simulink model "Model_RB_APF_WF_VO_withFairRules"  (R2024b)
settings: Solver=FixedStepAuto  StartTime=0.0  StopTime=150  FixedStep=UAVSampleTime  RelTol=1e-3
undefined symbols (not defined in the file): DroneMass, Gravity, Horizontal_Limits, Horizontal_Res, kD_pos, kD_vel, kI_pos, kI_vel, kP_pos, kP_vel, Lidar, MaxRange, N_filter, TopSpeed, UAV, Vertical_Limits, Vertical_Res, Waypoints
libraries: slpidlib x6, uavsimlib x4, robotcorelib x1, uavalgslib x1
(part 2 of 2)

== matlab function Model_RB_APF_WF_VO_withFairRules/LML Indicators/LML_indicators ==
  settings: updateMethod=DISCRETE
  data: APF_pos input; APF_mag output; position input; target input; disp_1s output; t input; disp_3s output; dist2goal output
function [APF_mag, disp_1s, disp_3s, dist2goal] = LML_indicators(APF_pos, position, target, t)

Tmax = 180;

persistent pos_hist
persistent lastSec

if isempty(pos_hist)
    pos_hist = zeros(Tmax+1, 3);
    lastSec  = int32(-1);
end

% APF_mag 
APF_mag = norm(APF_pos(:) - position(:));

% Time and Pos_hist
sec = int32(floor(t));
if sec ~= lastSec && sec >= 0 && sec <= Tmax
    pos_hist(sec+1, :) = position(:).';
    lastSec = sec;
end

% Disp1s
if sec >= 1
    disp_1s = norm(position(:) - pos_hist(sec, :).');
else
    disp_1s = 0;
end

% Disp3s
if sec >= 3
    disp_3s = norm(position(:) - pos_hist(sec-2, :).');
else
    disp_3s = 0;
end

% Dist2goal
dist2goal = norm(target-position);

== matlab function Model_RB_APF_WF_VO_withFairRules/Rule-Based Mode Switcher/RB mode manager ==
  settings: updateMethod=DISCRETE
  data: position input; flight_mode output; goal input; cloud input; APF_pos input; WF_pos input; t input; desired_pos output; Minima_list output; Minima_count output; critPoint_list output; critPoint_count output; LM_ind input; CP_ind input
function [flight_mode, desired_pos, Minima_list, Minima_count, critPoint_list, critPoint_count] = modeManager(position, goal, cloud, APF_pos, WF_pos, t, LM_ind, CP_ind)

% Parameters

thresh_F_APF        = 2;  
thresh_d_goal       = 8;   
thresh_d_1s         = 0.5;
thresh_d_3s         = 1;

thresh_APF_WF_angle = 25;
thresh_LM_dist      = 4;
thresh_C_obs        = 0.5;

LMmax            = 100;     % max VOs
CPmax                = 100;     % max CPs

% Persistent variables
persistent mode
persistent LM_list
persistent LM_count
persistent CP_list
persistent CP_count

if isempty(mode)
    mode             = 1;
    LM_list          = zeros(LMmax, 3);
    LM_count         = 0;
    CP_list          = zeros(CPmax, 3);
    CP_count         = 0;
end

% Unpack LM indicators
F_APF_mag    = LM_ind.F_APF_mag;
d_goal       = LM_ind.d_goal;
d_1s         = LM_ind.d_1s;
d_3s         = LM_ind.d_3s;

% Unpack CP indicators
theta_APF_WF = CP_ind.theta_APF_WF;
d_LM_closest = CP_ind.d_LM_closest;
C_obs        = CP_ind.C_obs;


% Default outputs
flight_mode    = mode;
desired_pos    = APF_pos;
Minima_list    = LM_list;
Minima_count   = LM_count;
critPoint_list  = CP_list;
critPoint_count = CP_count;

switch mode

    case 1  % APF mode

        desired_pos = APF_pos;

        force_is_weak   = F_APF_mag < thresh_F_APF;
        goal_is_close   = d_goal    < thresh_d_goal;
        barely_moved_1s = d_1s      < thresh_d_1s;
        barely_moved_3s = d_3s      < thresh_d_3s;

        LM_vote_force_goal = force_is_weak && ~goal_is_close;   % rules 1-4
        LM_vote_move_1s    = barely_moved_1s;                   % rules 5-6
        LM_vote_move_3s    = barely_moved_3s;                   % rules 7-8

        LM_votes = LM_vote_force_goal + LM_vote_move_1s + LM_vote_move_3s;

        if LM_votes >= 2   % LM trigger condition
            disp("Local Minima Detected at t ="); disp(t);
            
            % Place LM at current Position
            LM_count = LM_count + 1;
            LM_list(LM_count, :) = position(:).';
            assignin('base', 'finalMinimaList',  LM_list);
            assignin('base', 'finalMinimaCount', LM_count);

            % Determine WF direction (left or right)
            forwardXY    = goal(1:2) - position(1:2);
            left_points  = 0;
            right_points = 0;
            n_points = size(cloud, 1);
            for i = 1:n_points
                point_dir_XY = cloud(i, 1:2);
                cross_z = forwardXY(1)*point_dir_XY(2) - point_dir_XY(1)*forwardXY(2);
                if cross_z > 0
                    left_points = left_points + 1;
                elseif cross_z < 0
                    right_points = right_points + 1;
                end
            end
            if left_points < right_points
                mode = 2;
            else
                mode = 3;
            end
        end

        flight_mode = mode;
        Minima_list = LM_list;
        Minima_count = LM_count;

    case {2, 3}  % WF mode

        desired_pos = WF_pos;

        directions_aligned = theta_APF_WF < thresh_APF_WF_angle;
        near_LM            = d_LM_closest < thresh_LM_dist;
        area_is_open       = C_obs        < thresh_C_obs;

        CP_vote_angle   = directions_aligned;   % rules 1-2
        CP_vote_LM_dist = ~near_LM;             % rule 3 (two-sided: far from LM votes CP)
        CP_vote_density = area_is_open;         % rules 4-5

        CP_votes = CP_vote_angle + CP_vote_LM_dist + CP_vote_density;

        if CP_votes >= 2   % CP trigger condition
        
            CP_count = CP_count + 1;
            CP_list(CP_count, :) = position(:).';
            assignin('base', 'finalCPList',  CP_list);
            assignin('base', 'finalCPCount', CP_count);
            mode = 1;
        end

        flight_mode = mode;
        critPoint_list = CP_list;
        critPoint_count = CP_count;

    otherwise
        desired_pos = APF_pos;
        flight_mode = mode;
end

== matlab function Model_RB_APF_WF_VO_withFairRules/Controller/Attitude Control/Multirotor Acceleration Control ==
  data: acc input; roll output; pitch output; thrust output; yaw input; DroneMass parameter; Gravity parameter
function [roll, pitch, thrust] = accControl(acc, yaw, DroneMass, Gravity)

    xddot = acc(1);
    yddot = acc(2);
    zddot = acc(3);
    
    pitch = atan2((-xddot*cos(yaw)-yddot*sin(yaw)), ( -zddot + Gravity));
    roll = atan2(((-xddot*sin(yaw)+yddot*cos(yaw))*cos(pitch)), (-zddot+Gravity));
    
    roll_limit = 25*pi/180;
    pitch_limit = 25*pi/180;
    
    roll = min(roll_limit, max(-roll_limit, roll));
   
    pitch = min(pitch_limit, max(-pitch_limit, pitch));
    
    thrust = DroneMass*(-zddot+Gravity)/(cos(pitch)*cos(roll));
end

== matlab function Model_RB_APF_WF_VO_withFairRules/Path Planning Data/VOActivator_V5 ==
  settings: updateMethod=DISCRETE
  data: Minima_list input; Minima_count input; position input; Virtuals_list output; flight_mode input; Virtuals_count output; t input
function [Virtuals_list, Virtuals_count] = VOActivator(Minima_list, Minima_count, position, flight_mode, t)

activation_dist = 3;
maxVO = 100;

persistent VO_list
persistent VO_count
persistent next_to_check
persistent was_in_WF

if isempty(VO_list)
    VO_list      = zeros(maxVO, 3);
    VO_count     = 0;
    next_to_check = 1;
    was_in_WF     = false(maxVO, 1);

    % Pass to workspace at least once
    assignin('base', 'finalVOList',  VO_list);
    assignin('base', 'finalVOCount', VO_count);
    
end

% Mark all current unactivated minima as having been in WF
if flight_mode == 2 || flight_mode == 3
    was_in_WF(next_to_check:Minima_count) = true;
end

% Check unactivated minima for activation
for i = next_to_check:Minima_count
    d = norm(position(:) - Minima_list(i,:).');
    if d > activation_dist || (flight_mode == 1 && was_in_WF(i))
        % VO is activated
        %disp("VO Activated at t ="); disp(t);
        VO_count = VO_count + 1;
        VO_list(VO_count, :) = Minima_list(i,:);
        next_to_check = i + 1;
        % Update VO list in workspace
        assignin('base', 'finalVOList',  VO_list);
        assignin('base', 'finalVOCount', VO_count);
    end
end

Virtuals_list  = VO_list;
Virtuals_count = VO_count;

== matlab function Model_RB_APF_WF_VO_withFairRules/CPL Indicators/CPL_Indicators ==
  data: APF_pos input; APF_WF_ang output; WF_pos input; position input; Minima_list input; Minima_count input; cloud input; dist_closest_minima output; angular_coverage output
function [APF_WF_ang, dist_closest_minima, angular_coverage] = CPL_inputs(APF_pos, WF_pos, position, Minima_list, Minima_count, cloud)

% Parameters
max_dist = 10;
n_bins   = 36;

% APF_WF angle
APF_dir    = APF_pos(:) - position(:);
WF_dir     = WF_pos(:)  - position(:);
APF_WF_ang = rad2deg(acos(dot(APF_dir, WF_dir)/max(1e-6,(norm(APF_dir)*norm(WF_dir)))));

% Distance to closest minima
if Minima_count > 0
    diffs = Minima_list(1:Minima_count,:) - position(:).';
    dists = sqrt(sum(diffs.^2, 2));
    dist_closest_minima = min([min(dists(:)), max_dist]);
else
    dist_closest_minima = max_dist;
end

% Angular coverage

bearings = atan2(cloud(:,2), cloud(:,1));
bin_indices = mod(floor(bearings / (2*pi/n_bins)), n_bins) + 1;
bin_indices = max(1, min(n_bins, bin_indices));
bins = false(n_bins, 1);
bins(bin_indices) = true;
angular_coverage = sum(bins) / n_bins;
